simulink model "quarter_car_model"  (R2023b)
settings: Solver=VariableStepAuto  StartTime=0.0  StopTime=100  RelTol=1e-3
values from neighbouring files (symbols this model uses):
  c1 = 12    [data_small_racing_vehicle.m]
  k1 = 23    [data_small_racing_vehicle.m]
  k2 = 700    [data_small_racing_vehicle.m]
  mc = 60    [data_small_racing_vehicle.m]
  ms = 12    [data_small_racing_vehicle.m]
settings Model: Creator=NITRO  LastModifiedBy=NITRO

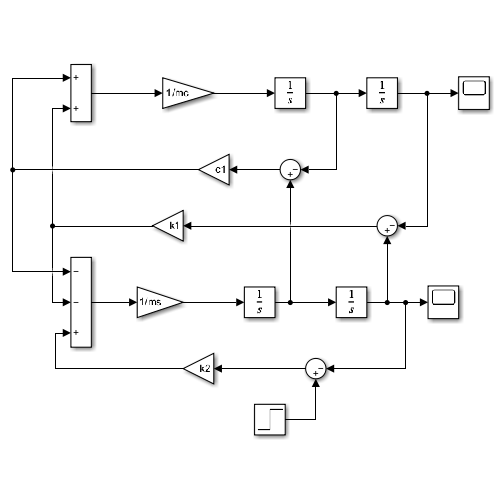
[thumbnail: Simulink's stored preview of the top-level diagram]
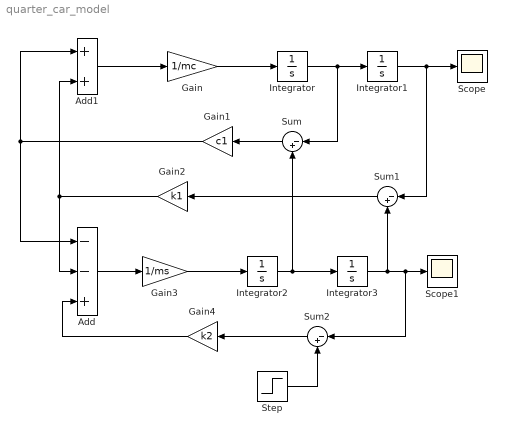
== system quarter_car_model ==
  Add : Sum  Inputs=--+
  Add1 : Sum
  Gain : Gain  Gain=1/mc
  Gain1 : Gain  Gain=c1
  Gain2 : Gain  Gain=k1
  Gain3 : Gain  Gain=1/ms
  Gain4 : Gain  Gain=k2
  Integrator{,1..3} (4 alike) : Integrator
  Scope : Scope
  Scope1 : Scope
  Step : Step  SampleTime=0
  Sum : Sum  Inputs=|-+
  Sum1 : Sum  Inputs=|-+
  Sum2 : Sum  Inputs=|-+
  wires:
  Add1/1 -> Gain/1
  Gain/1 -> Integrator/1
  Integrator/1 -> Sum/1, Integrator1/1
  Integrator1/1 -> Sum1/1, Scope/1
  Sum/1 -> Gain1/1
  Integrator3/1 -> Sum2/1, Scope1/1, Sum1/2
  Integrator2/1 -> Sum/2, Integrator3/1
  Gain3/1 -> Integrator2/1
  Sum1/1 -> Gain2/1
  Step/1 -> Sum2/2
  Sum2/1 -> Gain4/1
  Add/1 -> Gain3/1
  Gain4/1 -> Add/3
  Gain2/1 -> Add/2, Add1/2
  Gain1/1 -> Add1/1, Add/1
